simulink model "RC_RC_bipolar_vergl"  (R2013a)
settings: Solver=ode23  SolverMode=SingleTasking  StartTime=0.0  StopTime=50e-3  FixedStep=FS/50  MaxStep=1e-4  RelTol=1e-3
InitFcn:
  | %%%%%%  set scope time range
  | T_STOP=str2num(get_param(gcs,'StopTime'));
  | if numel(T_STOP) > 1
  |    T_STOP=T_STOP(2);
  | else
  |    T_STOP=T_STOP(1);
  | end
  | T_STOP=num2str(T_STOP);
  | 
  | %%%%%%  set scope time range in system @init_callback_fct
  | T_STOP=num2str(str2num(get_param(gcs,'StopTime')));
  | 
  | childs = allchild(0);
  | sol=strfind(upper(get(allchild(0),'Tag')),'VIEWER_PARAMETERS');
  | 
  | if iscell(sol)
  |    ind=find(~cellfun(@isempty, strfind(upper(get(allchild(0),'Tag')),'VIEWER_PARAMETERS')));
  | else
  |    ind=sol;
  | end
  | %ind=find(~cellfun(@isempty, {strfind(upper(get(allchild(0),'Tag')),'VIEWER_PARAMETERS'),[]}))
  | if ~isempty(ind)
  |    for k=1:length(childs(ind))
  |       set_param(getfield(get(childs(ind(k)),'UserData'),'block'),'TimeRange',T_STOP);
  |       get_param(getfield(get(childs(ind(k)),'UserData'),'block'),'TimeRange');
  | %    set_param(getfield(get(childs(ind),'UserData'),'block'),'TimeRange',T_STOP);
  | %    get_param(getfield(get(childs(ind),'UserData'),'block'),'TimeRange');
  |    end
  | else
  |     warning(sprintf('VIEWER_PARAMETERS object not found\nOpen the config dialog by hand for the first sim start'))
  | end
values from neighbouring files (symbols this model uses):
  FS = 5e-6    (= 5e-06)    [GalvoModel_v4_sys.m]    (also in GalvoModel_v6_sys.m = 5e-05; Galvo_process_analyze.m = 0.0001)
  Lc = 170e-6    (= 0.00017)    [GalvoModel_v6_sys.m]    (also in Galvo_process_analyze.m)
  Rc = 1.5    [GalvoModel_v6_sys.m]    (also in Galvo_process_analyze.m; frequenzgang_nichtinvert_opamp_koblitz_eas.m = 1)
  Rsh = 0.003    [GalvoModel_v6_sys.m]    (also in Galvo_sys_proto_v13_OFFSETS_MODEL_PT1B_proc.m = 0.075; frequenzgang_nichtinvert_opamp_koblitz_eas.m = 0.015)
  T1 = R1*C1    (= 0.000264)    [GalvoModel_v6_sys.m]
undefined symbols (not defined in the file or in its folder): CT1, RT1
libraries: simulink x1
settings Model: BufferReuse=off  Creator=mainster  LastModifiedBy=mainster
settings SolverCC: AutoInsertRateTranBlk=on
settings OptimizationCC: InlineParams=on  BufferReuse=off
settings DebuggingCC: InitInArrayFormatMsg=none
settings HardwareCC: ProdLargestAtomicInteger=Long  ProdLargestAtomicFloat=Double  ProdEndianess=LittleEndian  ProdHWDeviceType=ARM Compatible->ARM Cortex

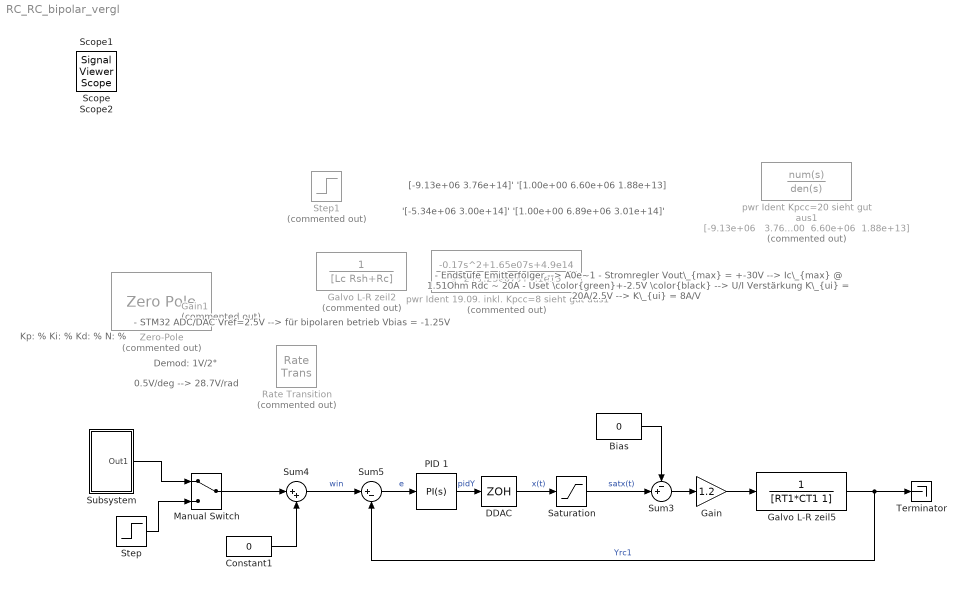
== system RC_RC_bipolar_vergl ==
  note: '[-5.34e+06 3.00e+14]' '[1.00e+00 6.89e+06 3.01e+14]'
  note: [-9.13e+06 3.76e+14]' '[1.00e+00 6.60e+06 1.88e+13]
  note: - Endstufe Emitterfolger --> A0e~1
      | - Stromregler Vout\_{max} = +-30V
      |       --> Ic\_{max} @ 1.51Ohm Rdc ~ 20A
      | - Uset \color{green}+-2.5V \color{black}
      |       --> U/I Verstärkung K\_{ui} = 20A/2.5V
      |       --> K\_{ui} = 8A/V
  note: - STM32 ADC/DAC Vref=2.5V
      | --> für bipolaren betrieb Vbias = -1.25V
  note: Kp: % Ki: % Kd: % N: %
  note: 0.5V/deg --> 28.7V/rad
  note: Demod:
      | 1V/2°
  Bias : Constant  Value=0  SampleTime=FS
  Constant1 : Constant  Value=0  SampleTime=0
  DDAC : ZeroOrderHold  SampleTime=FS
      settings: AttributesFormatString=%<SampleTime>
  Gain : Gain  Gain=1.2
  Gain1 : Gain  Commented=on  Gain=2
  Galvo L-R zeil2 : TransferFcn  Commented=on  Numerator=1  Denominator=[Lc Rsh+Rc]
  Galvo L-R zeil5 : TransferFcn  Numerator=1  Denominator=[RT1*CT1 1]
  Manual Switch : ManualSwitch  SampleTime=0
  PID 1 : simulink/Continuous/PID Controller  Controller=PI  TimeDomain=Continuous-time  SampleTime=0  IntegratorMethod=Forward Euler  FilterMethod=Forward Euler  Form=Parallel  P=10  I=0  D=9.0248898483108e-05  N=10930.7783722874  InitialConditionSource=internal  InitialConditionForIntegrator=0  InitialConditionForFilter=0  ExternalReset=none  LimitOutput=off  UpperSaturationLimit=1.25  LowerSaturationLimit=-1.25  LinearizeAsGain=on  AntiWindupMode=none  Kb=1  TrackingMode=off  Kt=1  PParamMin=[]  PParamMax=[]  IParamMin=[]  IParamMax=[]  DParamMin=[]  DParamMax=[]  NParamMin=[]  NParamMax=[]  KbParamMin=[]  KbParamMax=[]  KtParamMin=[]  KtParamMax=[]  POutMin=[]  POutMax=[]  IOutMin=[]  IOutMax=[]  DOutMin=[]  DOutMax=[]  NOutMin=[]  NOutMax=[]  KbOutMin=[]  KbOutMax=[]  KtOutMin=[]  KtOutMax=[]  IntegratorOutMin=[]  IntegratorOutMax=[]  FilterOutMin=[]  FilterOutMax=[]  SumOutMin=[]  SumOutMax=[]  SumI1OutMin=[]  SumI1OutMax=[]  SumI2OutMin=[]  SumI2OutMax=[]  SumI3OutMin=[]  SumI3OutMax=[]  SumDOutMin=[]  SumDOutMax=[]  SaturationOutMin=[]  SaturationOutMax=[]  IntegratorContinuousStateAttributes=''  IntegratorStateMustResolveToSignalObject=off  IntegratorRTWStateStorageClass=Auto  FilterContinuousStateAttributes=''  FilterStateMustResolveToSignalObject=off  FilterRTWStateStorageClass=Auto
      settings: AttributesFormatString=Kp=%<P>\nKi=%<I>
  Rate Transition : RateTransition  Commented=on  OutPortSampleTime=FS
  Saturation : Saturate  UpperLimit=3.5  LowerLimit=0  SampleTime=FS
      settings: AttributesFormatString=Up_lim=%<UpperLimit>\nLo_lim=%<LowerLimit>
  Step : Step  Time=1e-3  SampleTime=0
  Step1 : Step  Commented=on  SampleTime=0
  Subsystem : Subsystem  mask{dc=1.25}
      mask prompts: dc "enter dc offset"
      mask TypeOptions dc: Constant/Value
  Sum3 : Sum  Inputs=-+|  SampleTime=FS
  Sum4 : Sum  Inputs=|++  SampleTime=0
  Sum5 : Sum  Inputs=|+-  SampleTime=0
  Terminator : Terminator
  Zero-Pole : ZeroPole  Commented=on  Zeros=[]  Poles=[-1/T1 -1/T1]  Gain=(1/T1)^2
  pwr Ident 19.09. inkl. Kpcc=8 sieht gut aus1 : TransferFcn  Commented=on  Numerator=|  Denominator="[1  1.23e07  6.1e13]"
      | [-0.17  1.65e07  4.9e14
      | ]
  pwr Ident Kpcc=20 sieht gut aus1 : TransferFcn  Commented=on  Numerator="[-9.13e+06   3.76e+14]"  Denominator="[1.00e+00  6.60e+06  1.88e+13]"
  Scope : SignalViewerScope  IOType=viewer  NumInputPorts=3  RefreshTime=0.035000
      settings: ShowLegends=on  TimeRange=0.01  YMin=-5~-5~-5  YMax=5~5~5
  Scope1 : SignalViewerScope  IOType=viewer  LegendLocations="0.80742     0.84238     0.15391    0.089755"  RefreshTime=0.035000
      settings: ShowLegends=on  TimeRange=0.01
  Scope2 : SignalViewerScope  IOType=viewer  NumInputPorts=3  LegendLocations=|  RefreshTime=0.035000
      | 0.81988     0.93649     0.14149    0.049324
      | 0.81988     0.62189     0.15191    0.027027
      | 0.81988     0.30622     0.14149    0.049324
      settings: ShowLegends=on  TimeRange=0.05  YMin=0~-4~-1  YMax=2.5~12~2.5  SaveName=ScopeData2
  wires:
  Constant1/1 -> Sum4/2
  Sum4/1 -> Sum5/1  "win"
  Galvo L-R zeil5/1 -> Terminator/1, Sum5/2  "Yrc1"
  Sum5/1 -> PID 1/1  "e"
  Manual Switch/1 -> Sum4/1
  Step/1 -> Manual Switch/2
  Saturation/1 -> Sum3/2  "satx(t)"
  Bias/1 -> Sum3/1
  Sum3/1 -> Gain/1
  DDAC/1 -> Saturation/1  "x(t)"
  PID 1/1 -> DDAC/1  "pidY"
  Gain/1 -> Galvo L-R zeil5/1
  Subsystem/1(Out1) -> Manual Switch/1

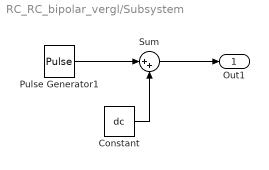
== system RC_RC_bipolar_vergl/Subsystem ==
  Constant : Constant  Value=dc
  Pulse Generator1 : DiscretePulseGenerator  PulseType=Time based  Period=10e-3  PulseWidth=50  SampleTime=0
  Sum : Sum  Inputs=|++
  Out1 : Outport
  wires:
  Pulse Generator1/1 -> Sum/1
  Constant/1 -> Sum/2
  Sum/1 -> Out1/1
